simulink model "simulator_v1_noRef"  (R2022b)
settings: Solver=ode8  StartTime=0.0  StopTime=simulation_time  FixedStep=dt  RelTol=1e-3
values from neighbouring files (symbols this model uses):
  automatic_control_enable = 0    [init_script.m]
  b = 9.17    [init_script.m]
  c = 2.15    [init_script.m]
  cg = 0.23    [init_script.m]
  cg_ref = 0.245    [init_script.m]
  cVect = [0 1 1+dt 8 8+dt simulation_time]    [init_script.m]
  deVect = [0 0 -0.02 -0.02 0 0]+dess    [init_script.m]
  m = 6000    [init_script.m]
  manual_control_enable = 0    [init_script.m]
  rho = 1.293    [init_script.m]
  s = 18.8    [init_script.m]
  theta_init = alpha_ss    [init_script.m]
  thrustss = []    [init_script.m]
  u_init = TAS_init*cos(alpha_ss)    [init_script.m]
  v_init = 0    [init_script.m]
  vector_control_enable = 1    [init_script.m]
  w_init = TAS_init*sin(alpha_ss)    [init_script.m]
undefined symbols (not defined in the file or in its folder): al_vec, cd_vec, cl_vec, cm_vec, cx_alfa, cyal_cagi, mz_alfa_cagi
libraries: shared6dof x1, simulink x1, aerolibanimutils x1
settings Model: Creator=lasto  LastModifiedBy=lasto

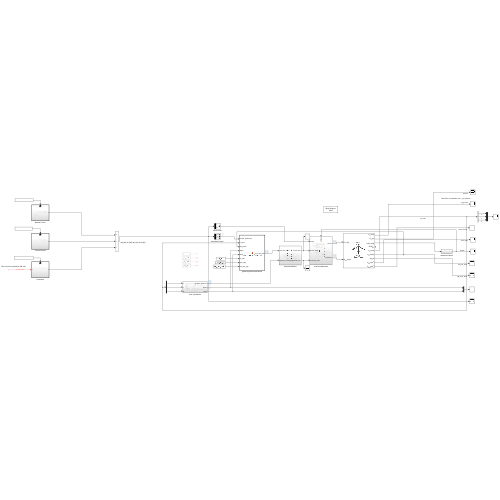
[thumbnail: Simulink's stored preview of the top-level diagram]
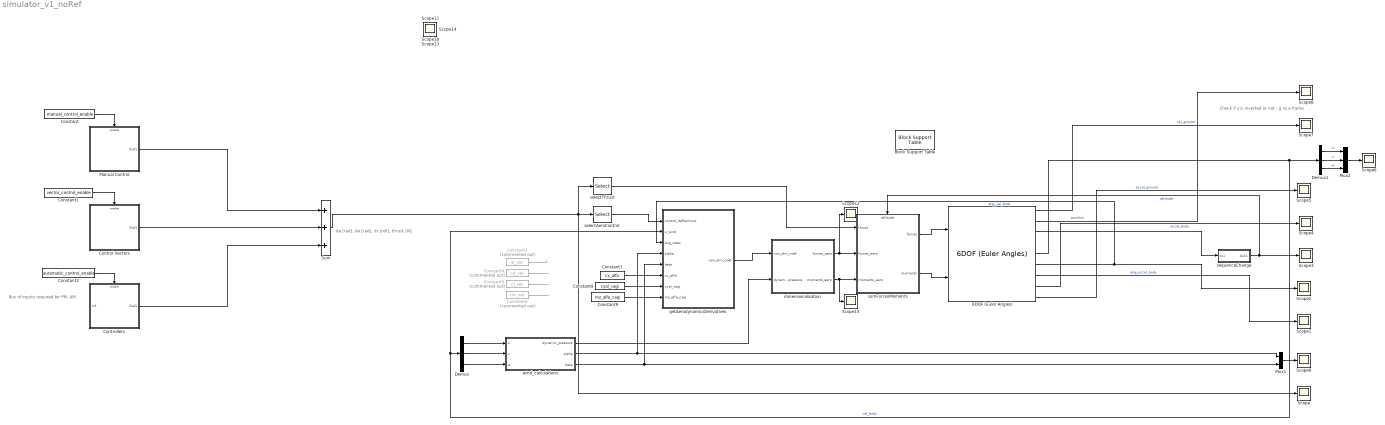
== system simulator_v1_noRef ==
  note: Check if z is inverted or not - g vs e frame
  note: da [rad], de [rad], dr [roll], thrust [N]
  note: Bus of inputs required for PM, AM
  6DOF (Euler Angles) : shared6dof/6DOF (Euler Angles)  units=Metric (MKS)  mtype=Fixed  rep=Euler Angles  xme_0=[0 0 0]  Vm_0=[u_init v_init w_init]  eul_0=[0 theta_init 0]  pm_0=[0 0 0]  mass_0=m  mass_e=0.5  mass_f=2.0  inertia=inertia  inertia_e=eye(3)  inertia_f=2*eye(3)  k_quat=1.0  vre_flag=on  abi_flag=on  aMode=0  xme_statename=''  Vm_statename=''  eul_statename=''  quat_statename=''  pm_statename=''  mass_statename=''
  Block Support Table : simulink/Model-Wide Utilities/Block Support Table
  Constant : Constant  Value=manual_control_enable
  Constant1 : Constant  Value=vector_control_enable
  Constant2 : Constant  Value=automatic_control_enable
  Constant3 : Constant  Commented=on  Value=al_vec
  Constant4 : Constant  Commented=on  Value=cd_vec
  Constant5 : Constant  Commented=on  Value=cl_vec
  Constant6 : Constant  Commented=on  Value=cm_vec
  Constant7 : Constant  Value=cx_alfa
  Constant8 : Constant  Value=cyal_cagi
  Constant9 : Constant  Value=mz_alfa_cagi
  Control Vectors : Subsystem
  Controllers : Subsystem
  Demux : Demux  Outputs=3
  Demux1 : Demux  Outputs=3
  Manual Control : Subsystem
  Mux1 : Mux  Inputs=2
  Mux2 : Mux  Inputs=3
  Scope{,1..15} (16 alike) : Scope
  Sum : Sum  Inputs=+++
  dimensionalisation : Subsystem
  getAerodynamicsDerivatives : MATLAB Function  TreatAsAtomicUnit=on
  selectAeroControl : Selector  InputPortWidth=4  IndexOptions=Index vector (dialog)  Indices=[1 2 3]  OutputSizes=1
  selectThrust : Selector  InputPortWidth=4  IndexOptions=Index vector (dialog)  Indices=[4]  OutputSizes=1
  sequenceChange : Subsystem
  sumForcesMoments : Subsystem
      settings: PortSchema="{\"entries\":[{\"content\":{\"sides\":[{\"content\":{\"connectorIds\":[\"In1\",\"In2\",\"In3\"]},\"type\":\"ConnectorPlacement.EquallySpacedRectSide\",\"uuid\":\"ac8242a7-5e4d-4a3c-9207-7fc263a49ce1\"},{\"content\":{\"connectorIds\":[\"Out1\",\"Out2\"],\"side\":\"RIGHT\"},\"type\":\"ConnectorPlacement.EquallySpacedRectSide\",\"uuid\":\"8b94f942-cff8-49a3-aa20-27e7cbd9c38a\"},{\"content\":{\"connectorIds\":[\"In4\"],\"side\":\"TOP\"},\"type\":\"ConnectorPlacement.EquallySpacedRectSide\",\"uuid\":\"879584ea-29a1-41c5-aa61-4afb24bb7a5f\"}]},\"type\":\"ConnectorPlacement.EquallySpacedConnector\",\"uuid\":\"af0172ac-4cc3-40fa-8ee6-f346b0b5a1a1\"}],\"packageUris\":[\"http://schema.mathworks.com/mf0/Connector/R2020b\"],\"version\":\"1.0\"}"
  wind_calculations : Subsystem
  wires:
  wind_calculations/1(dynamic_pressure) -> dimensionalisation/2(dynamic_pressure)
  Demux/2 -> wind_calculations/2(v)
  6DOF (Euler Angles)/9 -> Scope5/1  "accel_ground"
  Demux/1 -> wind_calculations/1(u)
  getAerodynamicsDerivatives/1(non_dim_coef) -> dimensionalisation/1(non_dim_coef)
  6DOF (Euler Angles)/2 -> Scope8/1  "position"
  sequenceChange/1(Out1) -> sumForcesMoments/4(attitude), Scope3/1  "attitude"
  Demux/3 -> wind_calculations/3(w)
  6DOF (Euler Angles)/7 -> Scope1/1  "ang_accel_body"
  dimensionalisation/1(forces_aero) -> Scope12/1, sumForcesMoments/2(forces_aero)
  6DOF (Euler Angles)/1 -> Scope7/1  "vel_ground"
  Sum/1 -> Scope/1, selectAeroControl/1, selectThrust/1
  6DOF (Euler Angles)/3 -> sequenceChange/1(In1)
  wind_calculations/2(alpha) -> Mux1/1, getAerodynamicsDerivatives/4(alpha)
  6DOF (Euler Angles)/6 -> Scope2/1, getAerodynamicsDerivatives/3(ang_rates)  "ang_vel_body"
  wind_calculations/3(beta) -> getAerodynamicsDerivatives/5(beta), Mux1/2
  sumForcesMoments/2(moments) -> 6DOF (Euler Angles)/2
  selectAeroControl/1 -> getAerodynamicsDerivatives/1(control_deflections)
  sumForcesMoments/1(forces) -> 6DOF (Euler Angles)/1
  6DOF (Euler Angles)/5 -> Demux1/1, getAerodynamicsDerivatives/2(v_wind), Demux/1  "vel_body"
  selectThrust/1 -> sumForcesMoments/1(thrust)
  dimensionalisation/2(moments_aero) -> Scope15/1, sumForcesMoments/3(moments_aero)
  6DOF (Euler Angles)/8 -> Scope4/1  "accel_body"
  Constant/1 -> Manual Control/Enable
  Controllers/1(Out1) -> Sum/3
  Constant2/1 -> Controllers/Enable
  ? -> Controllers/1(In1)
  Constant1/1 -> Control Vectors/Enable
  Manual Control/1(Out1) -> Sum/1
  Control Vectors/1(Out1) -> Sum/2
  Mux1/1 -> Scope9/1
  Demux1/1 -> Mux2/1  "u"
  Demux1/2 -> Mux2/2  "v"
  Demux1/3 -> Mux2/3  "w"
  Mux2/1 -> Scope6/1
  Constant3/1 -> ?
  Constant5/1 -> ?
  Constant4/1 -> ?
  Constant6/1 -> ?
  Constant7/1 -> getAerodynamicsDerivatives/6(cx_alfa)
  Constant9/1 -> getAerodynamicsDerivatives/8(mz_alfa_cagi)
  Constant8/1 -> getAerodynamicsDerivatives/7(cyal_cagi)

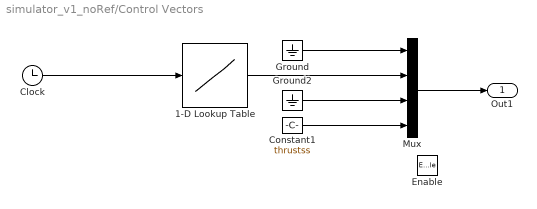
== system simulator_v1_noRef/Control Vectors ==
  Enable : EnablePort
  1-D Lookup Table : Lookup_n-D  NumberOfTableDimensions=1  BreakpointsForDimension1=cVect  Table=deVect  InternalRulePriority=Speed  RndMeth=Simplest
  Clock : Clock
  Constant1 : Constant  Value=thrustss
  Ground : Ground
  Ground2 : Ground
  Mux : Mux
  Out1 : Outport  OutputWhenDisabled=reset  InitialOutput=[0,0,0,0]
  wires:
  Mux/1 -> Out1/1
  1-D Lookup Table/1 -> Mux/2
  Ground/1 -> Mux/1
  Ground2/1 -> Mux/3
  Constant1/1 -> Mux/4
  Clock/1 -> 1-D Lookup Table/1

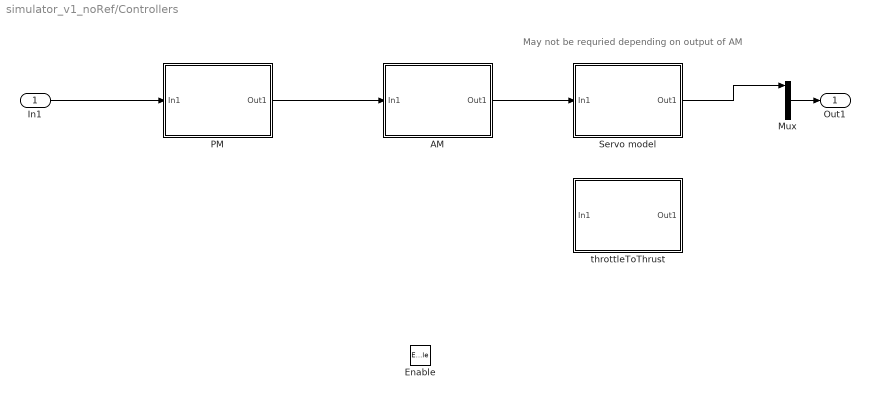
== system simulator_v1_noRef/Controllers ==
  note: May not be requried depending on output of AM
  In1 : Inport
  Enable : EnablePort
  AM : Subsystem
  Mux : Mux
  PM : Subsystem
  Servo model : Subsystem
  throttleToThrust : Subsystem
  Out1 : Outport  OutputWhenDisabled=reset  InitialOutput=[0,0,0,0]
  wires:
  In1/1 -> PM/1(In1)
  PM/1(Out1) -> AM/1(In1)
  AM/1(Out1) -> Servo model/1(In1)
  Servo model/1(Out1) -> Mux/1
  Mux/1 -> Out1/1

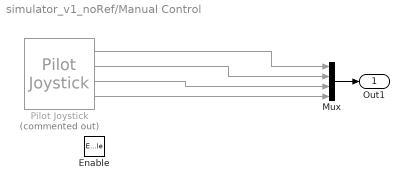
== system simulator_v1_noRef/Manual Control ==
  Enable : EnablePort
  Mux : Mux
  Pilot Joystick : aerolibanimutils/Pilot Joystick  Commented=on  JoystickID=Joystick1  OutputConfiguration=FourAxis  SampleTime=1/30
  Out1 : Outport  OutputWhenDisabled=reset  InitialOutput=[0,0,0,0]
  wires:
  Pilot Joystick/1 -> Mux/1
  Mux/1 -> Out1/1
  Pilot Joystick/2 -> Mux/2
  Pilot Joystick/3 -> Mux/3
  Pilot Joystick/4 -> Mux/4

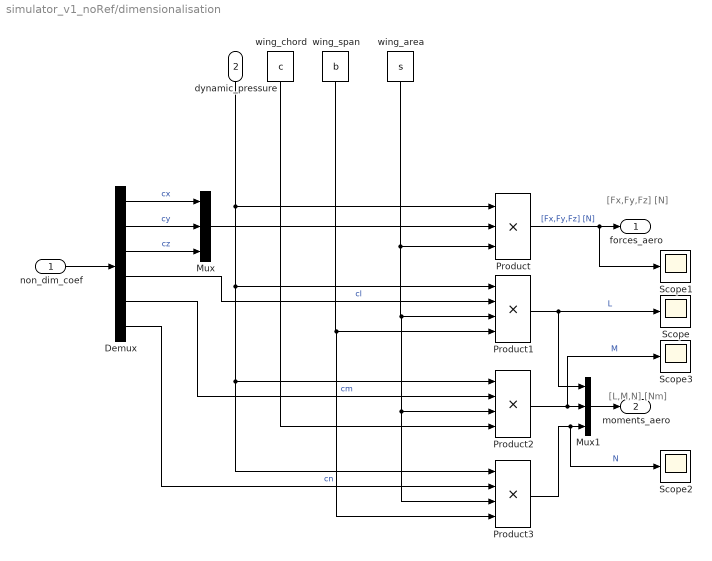
== system simulator_v1_noRef/dimensionalisation ==
  note: [L,M,N] [Nm]
  note: [Fx,Fy,Fz] [N]
  non_dim_coef : Inport
  dynamic_pressure : Inport  Port=2
  Demux : Demux  Outputs=6
  Mux : Mux  Inputs=3
  Mux1 : Mux  Inputs=3
  Product : Product  Inputs=3
  Product1 : Product  Inputs=4
  Product2 : Product  Inputs=4
  Product3 : Product  Inputs=4
  Scope{,1..3} (4 alike) : Scope
  wing_area : Constant  Value=s
  wing_chord : Constant  Value=c
  wing_span : Constant  Value=b
  forces_aero : Outport
  moments_aero : Outport  Port=2
  wires:
  non_dim_coef/1 -> Demux/1
  dynamic_pressure/1 -> Product1/1, Product3/1, Product2/1, Product/1
  Demux/6 -> Product3/2  "cn"
  Demux/5 -> Product2/2  "cm"
  Demux/4 -> Product1/2  "cl"
  Demux/3 -> Mux/3  "cz"
  Demux/2 -> Mux/2  "cy"
  Demux/1 -> Mux/1  "cx"
  Product/1 -> Scope1/1, forces_aero/1  "[Fx,Fy,Fz] [N]"
  Mux/1 -> Product/2
  wing_area/1 -> Product3/3, Product2/3, Product1/3, Product/3
  Mux1/1 -> moments_aero/1
  Product2/1 -> Scope3/1, Mux1/2  "M"
  Product3/1 -> Scope2/1, Mux1/3  "N"
  Product1/1 -> Scope/1, Mux1/1  "L"
  wing_span/1 -> Product3/4, Product1/4
  wing_chord/1 -> Product2/4

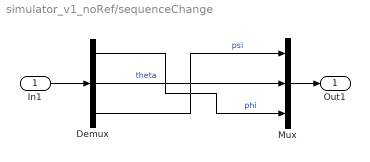
== system simulator_v1_noRef/sequenceChange ==
  In1 : Inport
  Demux : Demux  Outputs=3
  Mux : Mux  Inputs=3
  Out1 : Outport
  wires:
  In1/1 -> Demux/1
  Demux/3 -> Mux/1  "psi"
  Demux/2 -> Mux/2  "theta"
  Demux/1 -> Mux/3  "phi"
  Mux/1 -> Out1/1

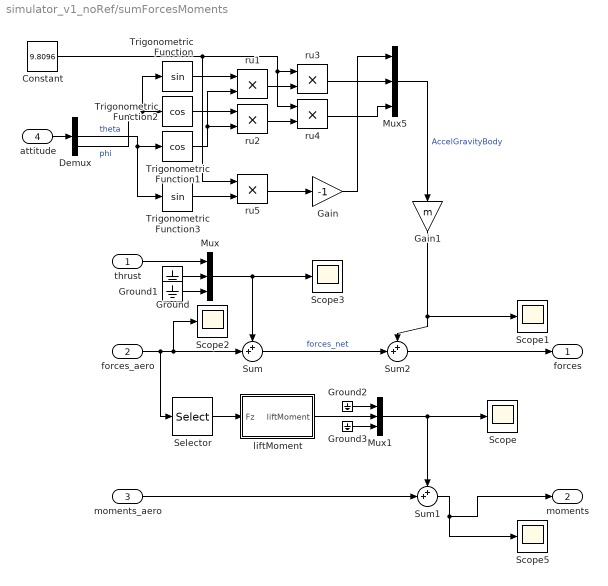
== system simulator_v1_noRef/sumForcesMoments ==
  thrust : Inport
  forces_aero : Inport  Port=2
  moments_aero : Inport  Port=3
  attitude : Inport  Port=4
  Constant : Constant  Value=9.8096
  Demux : Demux  Outputs=3
  Gain : Gain  Gain=-1
  Gain1 : Gain  Gain=m
  Ground{,1..3} (4 alike) : Ground
  Mux : Mux  Inputs=3
  Mux1 : Mux  Inputs=3
  Mux5 : Mux  Inputs=3
  Scope{,1..3,5} (5 alike) : Scope
  Selector : Selector  InputPortWidth=3  IndexOptions=Index vector (dialog)  Indices=[3]  OutputSizes=1
  Sum : Sum  Inputs=++|
  Sum1 : Sum  Inputs=++|
  Sum2 : Sum  Inputs=++|
  Trigonometric Function : Trigonometry
  Trigonometric Function1 : Trigonometry  Operator=cos
  Trigonometric Function2 : Trigonometry  Operator=cos
  Trigonometric Function3 : Trigonometry
  liftMoment : Subsystem
  ru{1..5} (5 alike) : Product  InputSameDT=on  SaturateOnIntegerOverflow=on  OutDataTypeStr=Inherit: Same as first input
  forces : Outport
  moments : Outport  Port=2
  wires:
  moments_aero/1 -> Sum1/2
  thrust/1 -> Mux/1
  Ground/1 -> Mux/2
  Ground1/1 -> Mux/3
  Sum/1 -> Sum2/2  "forces_net"
  Selector/1 -> liftMoment/1(Fz)
  Ground2/1 -> Mux1/1
  Ground3/1 -> Mux1/3
  Mux1/1 -> Scope/1, Sum1/1
  Trigonometric Function1/1 -> ru1/2, ru2/2
  Demux/2 -> Trigonometric Function1/1, Trigonometric Function3/1  "theta"
  ru3/1 -> Mux5/2
  Trigonometric Function/1 -> ru1/1
  Trigonometric Function3/1 -> ru5/2
  Mux5/1 -> Gain1/1  "AccelGravityBody"
  Constant/1 -> ru5/1, ru3/1, ru4/1
  ru4/1 -> Mux5/3
  ru2/1 -> ru4/2
  ru5/1 -> Gain/1
  ru1/1 -> ru3/2
  Gain/1 -> Mux5/1
  Demux/3 -> Trigonometric Function2/1, Trigonometric Function/1  "phi"
  Trigonometric Function2/1 -> ru2/1
  attitude/1 -> Demux/1
  Gain1/1 -> Scope1/1, Sum2/1
  forces_aero/1 -> Selector/1, Sum/2, Scope2/1
  Mux/1 -> Scope3/1, Sum/1
  liftMoment/1(liftMoment) -> Mux1/2
  Sum2/1 -> forces/1
  Sum1/1 -> moments/1, Scope5/1

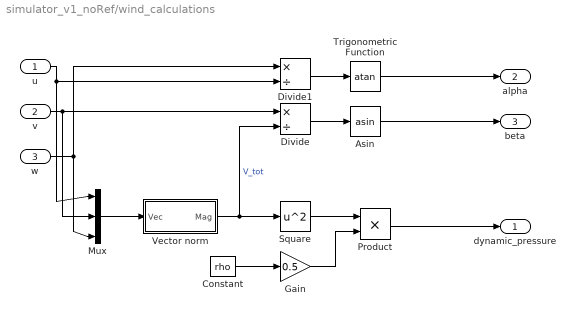
== system simulator_v1_noRef/wind_calculations ==
  u : Inport
  v : Inport  Port=2
  w : Inport  Port=3
  Asin : Trigonometry  Operator=asin
  Constant : Constant  Value=rho
  Divide : Product  Inputs=*/
  Divide1 : Product  Inputs=*/
  Gain : Gain  Gain=0.5
  Mux : Mux  Inputs=3
  Product : Product
  Square : Math  Operator=square
  Trigonometric Function : Trigonometry  Operator=atan
  Vector norm : Subsystem  mask(Vector norm-2){}
      mask help: Compute the 2-norm (magnitude) of a vector, |v| = sqrt(v'v).
      mask Help:
      | The block compute the 2-norm (or magnitude) of a vector.
      | <P><B>Input:</B> nx1 vector;</P>
      | <P><B>Output:</B> scalar magnitude.</P>
  dynamic_pressure : Outport
  alpha : Outport  Port=2
  beta : Outport  Port=3
  wires:
  u/1 -> Divide1/2, Mux/1
  v/1 -> Divide/1, Mux/2
  w/1 -> Divide1/1, Mux/3
  Mux/1 -> Vector norm/1(Vec)
  Vector norm/1(Mag) -> Divide/2, Square/1  "V_tot"
  Divide/1 -> Asin/1
  Asin/1 -> beta/1
  Divide1/1 -> Trigonometric Function/1
  Trigonometric Function/1 -> alpha/1
  Constant/1 -> Gain/1
  Square/1 -> Product/1
  Gain/1 -> Product/2
  Product/1 -> dynamic_pressure/1

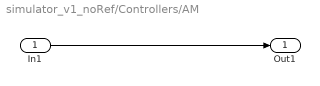
== system simulator_v1_noRef/Controllers/AM ==
  In1 : Inport
  Out1 : Outport
  wires:
  In1/1 -> Out1/1

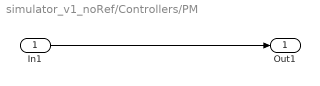
== system simulator_v1_noRef/Controllers/PM ==
  In1 : Inport
  Out1 : Outport
  wires:
  In1/1 -> Out1/1

== system simulator_v1_noRef/Controllers/Servo model ==
  In1 : Inport
  Out1 : Outport
  wires:
  In1/1 -> Out1/1

== system simulator_v1_noRef/Controllers/throttleToThrust ==
  In1 : Inport
  Out1 : Outport
  wires:
  In1/1 -> Out1/1

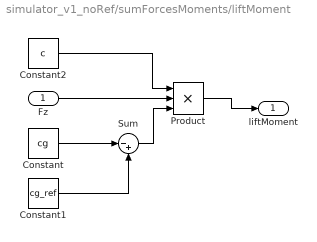
== system simulator_v1_noRef/sumForcesMoments/liftMoment ==
  Fz : Inport
  Constant : Constant  Value=cg
  Constant1 : Constant  Value=cg_ref
  Constant2 : Constant  Value=c
  Product : Product  Inputs=3
  Sum : Sum  Inputs=|-+
  liftMoment : Outport
  wires:
  Fz/1 -> Product/2
  Constant/1 -> Sum/1
  Constant1/1 -> Sum/2
  Sum/1 -> Product/3
  Product/1 -> liftMoment/1
  Constant2/1 -> Product/1

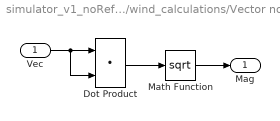
== system simulator_v1_noRef/wind_calculations/Vector norm ==
  Vec : Inport
  Dot Product : DotProduct  OutDataTypeStr=Inherit: Inherit via internal rule
  Math Function : Math  Operator=sqrt  SignedPower=on
  Mag : Outport
  wires:
  Dot Product/1 -> Math Function/1
  Vec/1 -> Dot Product/1, Dot Product/2
  Math Function/1 -> Mag/1

== matlab function simulator_v1_noRef/getAerodynamicsDerivatives ==
  data: control_deflections input; v_wind input; non_dim_coef output; ang_rates input; alpha input; beta input; cx_alfa input; cyal_cagi input; mz_alfa_cagi input
function non_dim_coef  = getAerodynamicDerivatives(control_deflections,v_wind,ang_rates,alpha,beta, cx_alfa, cyal_cagi, mz_alfa_cagi) %al_vec,cd_vec, cl_vec, cm_vec
% de = control_deflections(2);

% %% C172 
% cx0 = 0;
% cxu = -0.093; 
% cxalpha = 0.18;
% cxalphadot = 0; %likely wont be able to determine
% cxq = 0; 
% cxde = 0;  
% 
% czalpha = -4.631; 
% czalphadot = -0.850; %likely wont be able to determine
% czu = -0.620; 
% czq = -1.95;
% czde = -0.430;
% 
% cmalpha = -0.890;
% cmalphadot = -2.600; %likely wont be able to determine
% cmu = 0;
% cmq = -6.200;
% cmde = -1.28;
% 
% cx = cx0 + cxu + cxalpha*alpha + cxq*ang_rates(2) + cxde*control_deflections(2); % + *v_wind(1)
% cy = 0;
% cz = cz0 + czu + czalpha*alpha + czq*ang_rates(2) + czde*control_deflections(2); % + *v_wind(1)
% cl = 0;
% cm = cmalpha*alpha + cmu + cmq*ang_rates(2) + cmde*control_deflections(2);
% cn = 0;

%Set 2
% cm_al = -0.68;
% cl_al = 5.18;
% cm_q = -15.3;
% cl_q = 8.65;
% cl_de = 0.405;
% cm_de = -1.19;
% cr_be = -0.078;
% cr_p = -0.47;
% cr_r = 0.7;
% cr_da = -0.11;
% cr_dr = 0.0058;
% cn_be = 0.048;
% cn_p = -0.05;
% cn_r = -0.1;
% cn_da = -0.003;
% cn_dr = -0.053;
% cy_be = -0.59;
% cy_p = -0.045;
% cy_dr = 0.11;

% % Drag
% % CD = interp1(al_vec,cd_vec,alpha);
% 
% % Lift
% % CL = interp1(al_vec,cl_vec,alpha);
% 
% % Pitch moment
% % CM = interp1(al_vec,cm_vec,alpha) + cmde*de;
% 
% 
% %% Wind to body transformation
% CX0 = CL*sin(alpha)- CD*cos(alpha)*cos(beta);
% CY0 = -CD*sin(beta);
% CZ0 = (-CL*cos(alpha) - CD*cos(beta)*sin(alpha));
% 
% Cl0 = -CM*cos(alpha)*sin(beta);
% Cm0 =         CM*cos(beta);
% Cn0 = -CM*sin(alpha)*sin(beta);
% 
% non_dim_coef = [CX0,CY0,CZ0,Cl0,Cm0,Cn0];

% L159
da = control_deflections(1);
de = control_deflections(2);
dr = control_deflections(3);

V = norm(v_wind);
M = V/334.4; % at 5000ft

c = 2.15; 
b = 9.17;

p = ang_rates(1);
q = ang_rates(2);
r = ang_rates(3);
% adot = ABdot(1); ignore

deBuff = de;
if de > deg2rad(10) % Prevents extrapolation
    de = deg2rad(10);
end

alphaWingdeg = rad2deg(alpha)+2;

% Drag
CD = 0.03;

% Lift
CL = 0.22;

% Pitch moment
CM = 0.003-0.001*de;

%% X %%
Cxde = 0;
Cxq = 0;

%% Y %%
CYbeta = -1;         
Cyp = 0;
Cyr = 0;
CYda = -0.02;                                                  
CYdr = 0.192;

%% Z %%
Czalphadot = 0;
Czq = -1.45;

%% l %%
Clp = -0.41;
Clr = 0.13;
Clbeta = -0.08;
Clda = -0.14;
Cldr = 0.028;

%% m %%
Cmalphadot = -1.35;
Cmq = -4.9;

%% n %%
Cnp = 0.07;
Cnr = -0.4;
Cnbeta = 0.183;
Cnbetadot = 0;
Cnda = 0.001;                                                 
Cndr = -0.10;

%% Wind to body transformation
CX0 = CL*sin(alpha)- CD*cos(alpha)*cos(beta);
CY0 = -CD*sin(beta);
CZ0 = (-CL*cos(alpha) - CD*cos(beta)*sin(alpha));

Cl0 = -CM*cos(alpha)*sin(beta);
Cm0 =         CM*cos(beta);
Cn0 = -CM*sin(alpha)*sin(beta);

CX = CX0;                                              
CY = CY0 + CYbeta*beta + CYda*da + CYdr*dr;                                
CZ = CZ0 + c*q*Czq/V;
Cl = Cl0 + b*p*Clp/(2*V) + b*r*Clr/(2*V) + Clbeta*beta + Clda*da + Cldr*dr;
Cm = Cm0 + c*q*Cmq/V; % ignore c*adot*Cmalphadot/V;
Cn = Cn0 + Cnbeta*beta + b*p*Cnp/(2*V) + b*r*Cnr/(2*V) + Cnda*da + Cndr*dr;

non_dim_coef = [CX,CY,CZ,Cl,Cm,Cn];
end
